simulink model "SecRwRtStBkReclnHolderChk"  (R2018b)
settings: Solver=FixedStepDiscrete  StartTime=0.0  StopTime=10.0  FixedStep=0.01  RelTol=1e-3
libraries: simulink x4
settings Model: Creator=sn2xws  LastModifiedBy=sn2xws
settings Model: ModifiedHistory=|
  | 2023/11/7Bug 555794 童锁需要停止 21-26
  | 2024.5.8 V3.0.0 557 eze模式变更
  | 2024.9.9 V3.0.1 增加Md56
  | 2025.3.12 V3.8.0 bug 1002980 7s 调用mode 32和mode 53 ，调用过程中，等OTF展开后，二排靠背和三排靠背应同时展开
  | 25.7.7 V3.13.0 新增Md61 Md62
settings DataIOCC: SaveFormat=StructureWithTime
settings OptimizationCC: DefaultParameterBehavior=Inlined  EnhancedBackFolding=on  PassReuseOutputArgsAs=Individual arguments  ZeroExternalMemoryAtStartup=off  ZeroInternalMemoryAtStartup=off  OptimizeBlockOrder=speed  DifferentSizesBufferReuse=on  OptimizationCustomize=off
settings DebuggingCC: ParameterTunabilityLossMsg=error
settings ModelReferenceCC: ModelReferenceNumInstancesAllowed=Single
settings SFSimCC: MATLABDynamicMemAlloc=off
settings RTWCC: SystemTargetFile=autosar.tlc  GenCodeOnly=on  TemplateMakefile=ert_default_tmf  Description=AUTOSAR  GenerateReport=on  IncludeHyperlinkInReport=on  LaunchReport=on  GenerateTraceInfo=on  GenerateTraceReport=on  GenerateTraceReportSl=on  GenerateTraceReportSf=on  GenerateTraceReportEml=on
settings CodeAppCC: ForceParamTrailComments=on  IgnoreCustomStorageClasses=off  OperatorAnnotations=on  SimulinkDataObjDesc=on  SFDataObjDesc=on  InsertBlockDesc=on
settings STFCustomTargetCC: TargetLangStandard=C99 (ISO)  MultiwordLength=256  ParMdlRefBuildCompliant=on  CompOptLevelCompliant=on  IncludeMdlTerminateFcn=off  CombineOutputUpdateFcns=on  SuppressErrorStatus=on  ERTCustomFileBanners=on  SupportNonFinite=off  SupportComplex=off  SupportContinuousTime=off  SupportNonInlinedSFcns=off  RemoveResetFunc=on  MATLABClassNameForMDSCustomization=Simulink.SoftwareTarget.ERTCustomization  AutosarCompliant=on  UseToolchainInfoCompliant=on  LookupTableObjectStructAxisOrder=2,1,3,4,...  LUTObjectStructOrderEvenSpacing=Size,Table,Breakpoints  SystemTargetFile=autosar.tlc
settings ERTTargetCC: TargetLangStandard=C99 (ISO)  ConcurrentExecutionCompliant=off  IncludeMdlTerminateFcn=off  SuppressErrorStatus=on  SupportNonFinite=off  SupportComplex=off  ModelStepFunctionPrototypeControlCompliant=off  CPPClassGenCompliant=off  AutosarCompliant=on  LookupTableObjectStructAxisOrder=2,1,3,4,...  LUTObjectStructOrderEvenSpacing=Size,Table,Breakpoints  InlinedParameterPlacement=NonHierarchical  ERTCustomFileTemplate=example_file_process.tlc  ERTFilePackagingFormat=Compact

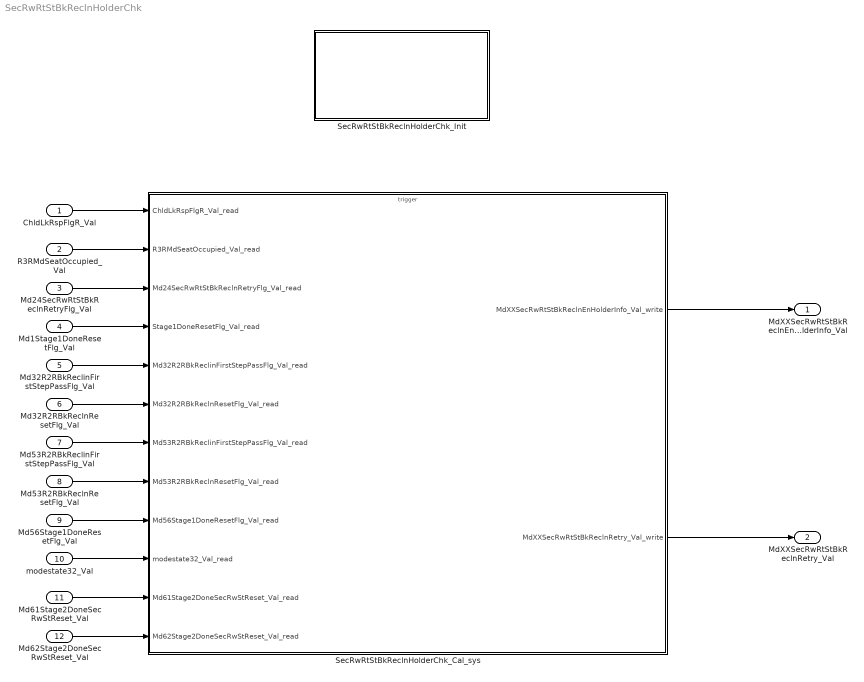
== system SecRwRtStBkReclnHolderChk ==
  ChldLkRspFlgR_Val : Inport  OutDataTypeStr=boolean  PortDimensions=1
  R3RMdSeatOccupied_Val : Inport  Port=2  OutDataTypeStr=boolean  PortDimensions=1
  Md24SecRwRtStBkReclnRetryFlg_Val : Inport  Port=3  OutDataTypeStr=boolean  PortDimensions=1
  Md1Stage1DoneResetFlg_Val : Inport  Port=4  OutDataTypeStr=boolean  PortDimensions=1
  Md32R2RBkReclinFirstStepPassFlg_Val : Inport  Port=5  OutDataTypeStr=boolean  PortDimensions=1
  Md32R2RBkReclnResetFlg_Val : Inport  Port=6  OutDataTypeStr=boolean  PortDimensions=1
  Md53R2RBkReclinFirstStepPassFlg_Val : Inport  Port=7  OutDataTypeStr=boolean  PortDimensions=1
  Md53R2RBkReclnResetFlg_Val : Inport  Port=8  OutDataTypeStr=boolean  PortDimensions=1
  Md56Stage1DoneResetFlg_Val : Inport  Port=9  OutDataTypeStr=boolean  PortDimensions=1
  modestate32_Val : Inport  Port=10  OutDataTypeStr=uint32  PortDimensions=1
  Md61Stage2DoneSecRwStReset_Val : Inport  Port=11  OutDataTypeStr=boolean  PortDimensions=1
  Md62Stage2DoneSecRwStReset_Val : Inport  Port=12  OutDataTypeStr=boolean  PortDimensions=1
  SecRwRtStBkReclnHolderChk_Cal_sys : Subsystem
  SecRwRtStBkReclnHolderChk_Init : Subsystem
  MdXXSecRwRtStBkReclnEnHolderInfo_Val : Outport  OutDataTypeStr=uint32  PortDimensions=1
  MdXXSecRwRtStBkReclnRetry_Val : Outport  Port=2  OutDataTypeStr=uint32  PortDimensions=1
  wires:
  ChldLkRspFlgR_Val/1 -> SecRwRtStBkReclnHolderChk_Cal_sys/1(ChldLkRspFlgR_Val_read)
  R3RMdSeatOccupied_Val/1 -> SecRwRtStBkReclnHolderChk_Cal_sys/2(R3RMdSeatOccupied_Val_read)
  SecRwRtStBkReclnHolderChk_Cal_sys/1(MdXXSecRwRtStBkReclnEnHolderInfo_Val_write) -> MdXXSecRwRtStBkReclnEnHolderInfo_Val/1
  Md24SecRwRtStBkReclnRetryFlg_Val/1 -> SecRwRtStBkReclnHolderChk_Cal_sys/3(Md24SecRwRtStBkReclnRetryFlg_Val_read)
  SecRwRtStBkReclnHolderChk_Cal_sys/2(MdXXSecRwRtStBkReclnRetry_Val_write) -> MdXXSecRwRtStBkReclnRetry_Val/1
  Md1Stage1DoneResetFlg_Val/1 -> SecRwRtStBkReclnHolderChk_Cal_sys/4(Stage1DoneResetFlg_Val_read)
  Md32R2RBkReclinFirstStepPassFlg_Val/1 -> SecRwRtStBkReclnHolderChk_Cal_sys/5(Md32R2RBkReclinFirstStepPassFlg_Val_read)
  Md32R2RBkReclnResetFlg_Val/1 -> SecRwRtStBkReclnHolderChk_Cal_sys/6(Md32R2RBkReclnResetFlg_Val_read)
  Md53R2RBkReclinFirstStepPassFlg_Val/1 -> SecRwRtStBkReclnHolderChk_Cal_sys/7(Md53R2RBkReclinFirstStepPassFlg_Val_read)
  Md53R2RBkReclnResetFlg_Val/1 -> SecRwRtStBkReclnHolderChk_Cal_sys/8(Md53R2RBkReclnResetFlg_Val_read)
  Md56Stage1DoneResetFlg_Val/1 -> SecRwRtStBkReclnHolderChk_Cal_sys/9(Md56Stage1DoneResetFlg_Val_read)
  modestate32_Val/1 -> SecRwRtStBkReclnHolderChk_Cal_sys/10(modestate32_Val_read)
  Md61Stage2DoneSecRwStReset_Val/1 -> SecRwRtStBkReclnHolderChk_Cal_sys/11(Md61Stage2DoneSecRwStReset_Val_read)
  Md62Stage2DoneSecRwStReset_Val/1 -> SecRwRtStBkReclnHolderChk_Cal_sys/12(Md62Stage2DoneSecRwStReset_Val_read)

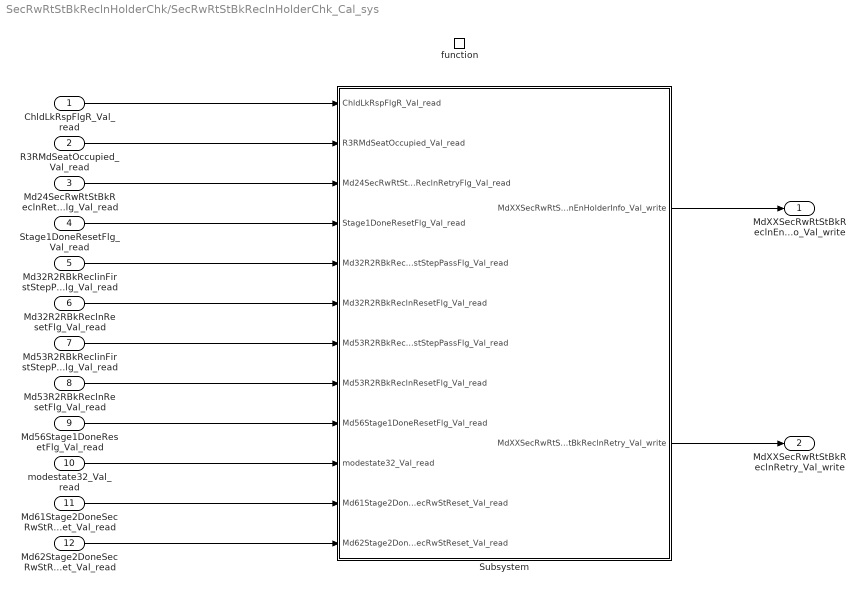
== system SecRwRtStBkReclnHolderChk/SecRwRtStBkReclnHolderChk_Cal_sys ==
  ChldLkRspFlgR_Val_read : Inport
  R3RMdSeatOccupied_Val_read : Inport  Port=2
  Md24SecRwRtStBkReclnRetryFlg_Val_read : Inport  Port=3
  Stage1DoneResetFlg_Val_read : Inport  Port=4
  Md32R2RBkReclinFirstStepPassFlg_Val_read : Inport  Port=5
  Md32R2RBkReclnResetFlg_Val_read : Inport  Port=6
  Md53R2RBkReclinFirstStepPassFlg_Val_read : Inport  Port=7
  Md53R2RBkReclnResetFlg_Val_read : Inport  Port=8
  Md56Stage1DoneResetFlg_Val_read : Inport  Port=9
  modestate32_Val_read : Inport  Port=10
  Md61Stage2DoneSecRwStReset_Val_read : Inport  Port=11
  Md62Stage2DoneSecRwStReset_Val_read : Inport  Port=12
  function : TriggerPort  TriggerType=function-call  IsSimulinkFunction=on  FunctionName=SecRwRtStBkReclnHolderChk_Cal  VariantControl=(inherit)
  Subsystem : Subsystem
  MdXXSecRwRtStBkReclnEnHolderInfo_Val_write : Outport
      settings: EnsureOutportIsVirtual=on
  MdXXSecRwRtStBkReclnRetry_Val_write : Outport  Port=2
      settings: EnsureOutportIsVirtual=on
  wires:
  Subsystem/1(MdXXSecRwRtStBkReclnEnHolderInfo_Val_write) -> MdXXSecRwRtStBkReclnEnHolderInfo_Val_write/1
  R3RMdSeatOccupied_Val_read/1 -> Subsystem/2(R3RMdSeatOccupied_Val_read)
  ChldLkRspFlgR_Val_read/1 -> Subsystem/1(ChldLkRspFlgR_Val_read)
  Md24SecRwRtStBkReclnRetryFlg_Val_read/1 -> Subsystem/3(Md24SecRwRtStBkReclnRetryFlg_Val_read)
  Subsystem/2(MdXXSecRwRtStBkReclnRetry_Val_write) -> MdXXSecRwRtStBkReclnRetry_Val_write/1
  Stage1DoneResetFlg_Val_read/1 -> Subsystem/4(Stage1DoneResetFlg_Val_read)
  Md53R2RBkReclinFirstStepPassFlg_Val_read/1 -> Subsystem/7(Md53R2RBkReclinFirstStepPassFlg_Val_read)
  Md53R2RBkReclnResetFlg_Val_read/1 -> Subsystem/8(Md53R2RBkReclnResetFlg_Val_read)
  Md32R2RBkReclinFirstStepPassFlg_Val_read/1 -> Subsystem/5(Md32R2RBkReclinFirstStepPassFlg_Val_read)
  Md32R2RBkReclnResetFlg_Val_read/1 -> Subsystem/6(Md32R2RBkReclnResetFlg_Val_read)
  Md56Stage1DoneResetFlg_Val_read/1 -> Subsystem/9(Md56Stage1DoneResetFlg_Val_read)
  modestate32_Val_read/1 -> Subsystem/10(modestate32_Val_read)
  Md61Stage2DoneSecRwStReset_Val_read/1 -> Subsystem/11(Md61Stage2DoneSecRwStReset_Val_read)
  Md62Stage2DoneSecRwStReset_Val_read/1 -> Subsystem/12(Md62Stage2DoneSecRwStReset_Val_read)

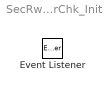
== system SecRwRtStBkReclnHolderChk/SecRwRtStBkReclnHolderChk_Init ==
  Event Listener : EventListener  EventName=reset

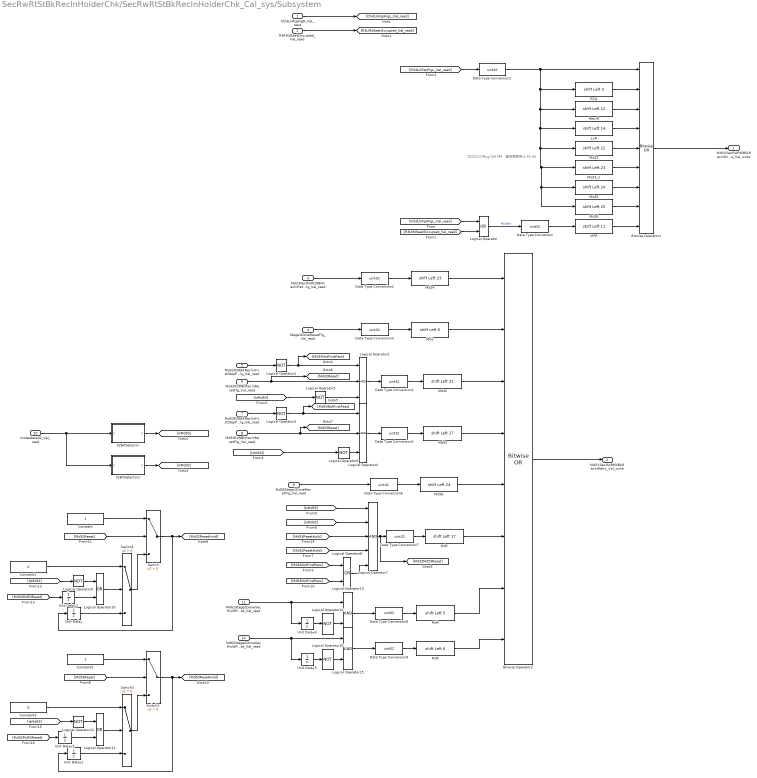
== system SecRwRtStBkReclnHolderChk/SecRwRtStBkReclnHolderChk_Cal_sys/Subsystem ==
  note: 2023/11/7Bug 555794 童锁需要停止 21-26
  ChldLkRspFlgR_Val_read : Inport
  R3RMdSeatOccupied_Val_read : Inport  Port=2
  Md24SecRwRtStBkReclnRetryFlg_Val_read : Inport  Port=3
  Stage1DoneResetFlg_Val_read : Inport  Port=4
  Md32R2RBkReclinFirstStepPassFlg_Val_read : Inport  Port=5
  Md32R2RBkReclnResetFlg_Val_read : Inport  Port=6
  Md53R2RBkReclinFirstStepPassFlg_Val_read : Inport  Port=7
  Md53R2RBkReclnResetFlg_Val_read : Inport  Port=8
  Md56Stage1DoneResetFlg_Val_read : Inport  Port=9
  modestate32_Val_read : Inport  Port=10
  Md61Stage2DoneSecRwStReset_Val_read : Inport  Port=11
  Md62Stage2DoneSecRwStReset_Val_read : Inport  Port=12
  32BitSelector : Subsystem  mask(32 Bit Selector){BitNum=17}
      mask prompts: BitNum "Select Bit Number"
      mask help: Allows selection of a particular bit (0-31) out of a packed word up to 32 bits long. Output will be true if the bit number selected via the mask parameter is equal to one.
      mask TypeOptions BitNum: 0 | 1 | 2 | 3 | 4 | 5 | 6 | 7 | 8 | 9 | 10 | 11 | 12 | 13 | 14 | 15 | 16 | 17 | 18 | 19 | 20 | 21 | 22 | 23 | 24 | 25 | 26 | 27 | 28 | 29 | 30 | 31
      mask Display:
      | text(0.5, 0.8,'BIT','horizontalAlignment','center')
      | text(0.5, 0.5,'SELECTOR','horizontalAlignment','center')
      | text(0.5, 0.2,['-- Bit ',char(get_param(gcb,'BitNum')),' --'],'horizontalAlignment','center')
  32BitSelector1 : Subsystem  mask(32 Bit Selector){BitNum=31}
      mask prompts: BitNum "Select Bit Number"
      mask help: Allows selection of a particular bit (0-31) out of a packed word up to 32 bits long. Output will be true if the bit number selected via the mask parameter is equal to one.
      mask TypeOptions BitNum: 0 | 1 | 2 | 3 | 4 | 5 | 6 | 7 | 8 | 9 | 10 | 11 | 12 | 13 | 14 | 15 | 16 | 17 | 18 | 19 | 20 | 21 | 22 | 23 | 24 | 25 | 26 | 27 | 28 | 29 | 30 | 31
      mask Display:
      | text(0.5, 0.8,'BIT','horizontalAlignment','center')
      | text(0.5, 0.5,'SELECTOR','horizontalAlignment','center')
      | text(0.5, 0.2,['-- Bit ',char(get_param(gcb,'BitNum')),' --'],'horizontalAlignment','center')
  Bitwise Operator1 : simulink/Logic and Bit Operations/Bitwise Operator  logicop=OR  UseBitMask=off  NumInputPorts=9  BitMask=bin2dec('11011001')  BitMaskRealWorld=Stored Integer
  Bitwise Operator2 : simulink/Logic and Bit Operations/Bitwise Operator  logicop=OR  UseBitMask=off  NumInputPorts=8  BitMask=bin2dec('11011001')  BitMaskRealWorld=Stored Integer
  Constant : Constant  OutDataTypeStr=boolean
  Constant1 : Constant  Value=0  OutDataTypeStr=boolean
  Constant2 : Constant  OutDataTypeStr=boolean
  Constant3 : Constant  Value=0  OutDataTypeStr=boolean
  Data Type Conversion{,1..9} (10 alike) : DataTypeConversion  OutDataTypeStr=uint32
  EZQ : ArithShift  BitShiftNumber=3  BitShiftDirection=Left
  Logical Operator{,8,10..11} (4 alike) : Logic  Operator=OR  AllPortsSameDT=off  OutDataTypeStr=boolean
  Logical Operator{1,3,5..6,9,12,14,16} (8 alike) : Logic  Operator=NOT  AllPortsSameDT=off  OutDataTypeStr=boolean
  Logical Operator13 : Logic  AllPortsSameDT=off  OutDataTypeStr=boolean
  Logical Operator15 : Logic  AllPortsSameDT=off  OutDataTypeStr=boolean
  Logical Operator2 : Logic  Inputs=3  AllPortsSameDT=off  OutDataTypeStr=boolean
  Logical Operator4 : Logic  Inputs=3  AllPortsSameDT=off  OutDataTypeStr=boolean
  Logical Operator7 : Logic  Inputs=5  AllPortsSameDT=off  OutDataTypeStr=boolean
  LyR : ArithShift  BitShiftNumber=14  BitShiftDirection=Left
  Md1 : ArithShift  BitShiftDirection=Left
  Md2 : ArithShift  BitShiftNumber=17  BitShiftDirection=Left
  Md23 : ArithShift  BitShiftNumber=22  BitShiftDirection=Left
  Md24 : ArithShift  BitShiftNumber=23  BitShiftDirection=Left
  Md24_2 : ArithShift  BitShiftNumber=23  BitShiftDirection=Left
  Md25 : ArithShift  BitShiftNumber=24  BitShiftDirection=Left
  Md26 : ArithShift  BitShiftNumber=25  BitShiftDirection=Left
  Md32 : ArithShift  BitShiftNumber=31  BitShiftDirection=Left
  Md4 : ArithShift  BitShiftNumber=5  BitShiftDirection=Left
  Md5 : ArithShift  BitShiftNumber=6  BitShiftDirection=Left
  Md53 : ArithShift  BitShiftNumber=17  BitShiftDirection=Left
  Md56 : ArithShift  BitShiftNumber=24  BitShiftDirection=Left
  RecvR : ArithShift  BitShiftNumber=12  BitShiftDirection=Left
  Switch{,1..3} (4 alike) : Switch  Criteria=u2 > Threshold
  Unit Delay{,1..5} (6 alike) : UnitDelay  SampleTime=-1
  VIPR : ArithShift  BitShiftNumber=11  BitShiftDirection=Left
  MdXXSecRwRtStBkReclnEnHolderInfo_Val_write : Outport
      settings: EnsureOutportIsVirtual=on
  MdXXSecRwRtStBkReclnRetry_Val_write : Outport  Port=2
      settings: EnsureOutportIsVirtual=on
  wires:
  [ChldLkRspFlgL_Val_read] -> Data Type Conversion1/1
  Bitwise Operator1/1 -> MdXXSecRwRtStBkReclnEnHolderInfo_Val_write/1
  LyR/1 -> Bitwise Operator1/4
  RecvR/1 -> Bitwise Operator1/3
  Logical Operator/1 -> Data Type Conversion/1  "Holder"
  Data Type Conversion/1 -> VIPR/1
  R3RMdSeatOccupied_Val_read/1 -> [R3LMdSeatOccupied_Val_read]
  Data Type Conversion1/1 -> Md26/1, Md25/1, Md24_2/1, Md23/1, LyR/1, RecvR/1, EZQ/1, Bitwise Operator1/1
  [ChldLkRspFlgL_Val_read] -> Logical Operator/1
  EZQ/1 -> Bitwise Operator1/2
  [R3LMdSeatOccupied_Val_read] -> Logical Operator/2
  ChldLkRspFlgR_Val_read/1 -> [ChldLkRspFlgL_Val_read]
  Md24SecRwRtStBkReclnRetryFlg_Val_read/1 -> Data Type Conversion2/1
  Data Type Conversion2/1 -> Md24/1
  VIPR/1 -> Bitwise Operator1/9
  Md23/1 -> Bitwise Operator1/5
  Md24_2/1 -> Bitwise Operator1/6
  Md25/1 -> Bitwise Operator1/7
  Md26/1 -> Bitwise Operator1/8
  Stage1DoneResetFlg_Val_read/1 -> Data Type Conversion3/1
  Data Type Conversion3/1 -> Md1/1
  Bitwise Operator2/1 -> MdXXSecRwRtStBkReclnRetry_Val_write/1
  Md24/1 -> Bitwise Operator2/1
  Md1/1 -> Bitwise Operator2/2
  Md32R2RBkReclinFirstStepPassFlg_Val_read/1 -> Logical Operator1/1
  Logical Operator1/1 -> [Md32NotFirstPass], Logical Operator2/1
  Md32R2RBkReclnResetFlg_Val_read/1 -> Logical Operator2/2, [Md32Reset]
  Logical Operator2/1 -> Data Type Conversion4/1
  Data Type Conversion4/1 -> Md32/1
  Md32/1 -> Bitwise Operator2/3
  Md53/1 -> Bitwise Operator2/4
  Data Type Conversion5/1 -> Md53/1
  Logical Operator4/1 -> Data Type Conversion5/1
  Md53R2RBkReclnResetFlg_Val_read/1 -> Logical Operator4/2, [Md53Reset]
  Logical Operator3/1 -> [Md53NotFirstPass], Logical Operator4/1
  Md53R2RBkReclinFirstStepPassFlg_Val_read/1 -> Logical Operator3/1
  Md56/1 -> Bitwise Operator2/5
  Data Type Conversion6/1 -> Md56/1
  Md56Stage1DoneResetFlg_Val_read/1 -> Data Type Conversion6/1
  32BitSelector/1(y) -> [IsMd53]
  32BitSelector1/1(y) -> [IsMd32]
  [IsMd53] -> Logical Operator5/1
  Logical Operator5/1 -> Logical Operator2/3
  [IsMd32] -> Logical Operator6/1
  Logical Operator6/1 -> Logical Operator4/3
  [IsMd53] -> Logical Operator7/1
  [IsMd32] -> Logical Operator7/2
  [Md32NotFirstPass] -> Logical Operator8/1
  [Md53NotFirstPass] -> Logical Operator8/2
  Logical Operator8/1 -> Logical Operator7/5
  Logical Operator7/1 -> [Md32Md53Reset], Data Type Conversion7/1
  modestate32_Val_read/1 -> 32BitSelector1/1(x), 32BitSelector/1(x)
  Data Type Conversion7/1 -> Md2/1
  Md2/1 -> Bitwise Operator2/6
  [Md32Reset] -> Switch/2
  Constant/1 -> Switch/1
  Switch/1 -> Unit Delay/1, [Md32ResetHold]
  Switch1/1 -> Switch/3
  [IsMd32] -> Logical Operator9/1
  Constant1/1 -> Switch1/1
  Logical Operator9/1 -> Logical Operator10/1
  [Md32Md53Reset] -> Unit Delay2/1
  Logical Operator10/1 -> Switch1/2
  Unit Delay/1 -> Switch1/3
  [Md32ResetHold] -> Logical Operator7/4
  Unit Delay1/1 -> Switch3/3
  Logical Operator11/1 -> Switch3/2
  [Md32Md53Reset] -> Unit Delay3/1
  Logical Operator12/1 -> Logical Operator11/1
  Constant3/1 -> Switch3/1
  [IsMd53] -> Logical Operator12/1
  Switch3/1 -> Switch2/3
  Switch2/1 -> [Md53ResetHold], Unit Delay1/1
  Constant2/1 -> Switch2/1
  [Md53Reset] -> Switch2/2
  [Md53ResetHold] -> Logical Operator7/3
  Unit Delay2/1 -> Logical Operator10/2
  Unit Delay3/1 -> Logical Operator11/2
  Data Type Conversion9/1 -> Md5/1
  Logical Operator15/1 -> Data Type Conversion9/1
  Logical Operator16/1 -> Logical Operator15/2
  Unit Delay4/1 -> Logical Operator14/1
  Md5/1 -> Bitwise Operator2/8
  Md4/1 -> Bitwise Operator2/7
  Logical Operator13/1 -> Data Type Conversion8/1
  Logical Operator14/1 -> Logical Operator13/2
  Unit Delay5/1 -> Logical Operator16/1
  Md62Stage2DoneSecRwStReset_Val_read/1 -> Logical Operator15/1, Unit Delay5/1
  Md61Stage2DoneSecRwStReset_Val_read/1 -> Logical Operator13/1, Unit Delay4/1
  Data Type Conversion8/1 -> Md4/1

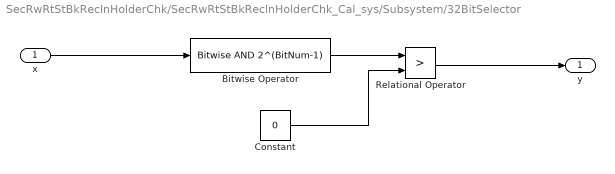
== system SecRwRtStBkReclnHolderChk/SecRwRtStBkReclnHolderChk_Cal_sys/Subsystem/32BitSelector ==
  x : Inport
  Bitwise Operator : simulink/Logic and Bit Operations/Bitwise Operator  logicop=AND  UseBitMask=on  BitMask=2^(BitNum-1)  BitMaskRealWorld=Stored Integer
  Constant : Constant  Value=0  OutDataTypeStr=uint32
  Relational Operator : RelationalOperator  Operator=>  OutDataTypeStr=boolean  RndMeth=Simplest
  y : Outport
  wires:
  Relational Operator/1 -> y/1
  Constant/1 -> Relational Operator/2
  x/1 -> Bitwise Operator/1
  Bitwise Operator/1 -> Relational Operator/1

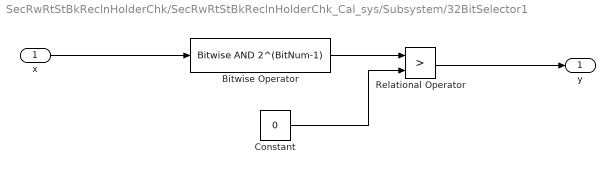
== system SecRwRtStBkReclnHolderChk/SecRwRtStBkReclnHolderChk_Cal_sys/Subsystem/32BitSelector1 ==
  x : Inport
  Bitwise Operator : simulink/Logic and Bit Operations/Bitwise Operator  logicop=AND  UseBitMask=on  BitMask=2^(BitNum-1)  BitMaskRealWorld=Stored Integer
  Constant : Constant  Value=0  OutDataTypeStr=uint32
  Relational Operator : RelationalOperator  Operator=>  OutDataTypeStr=boolean  RndMeth=Simplest
  y : Outport
  wires:
  Bitwise Operator/1 -> Relational Operator/1
  x/1 -> Bitwise Operator/1
  Constant/1 -> Relational Operator/2
  Relational Operator/1 -> y/1
